simulink library "discreteGainScheduledFilteredPID"  (R2022a)
settings: Solver=VariableStepAuto  StartTime=0.0  StopTime=10.0  RelTol=1e-3
undefined symbols (not defined in the file): Ts
settings Model: Creator=adabney  LastModifiedBy=jacob

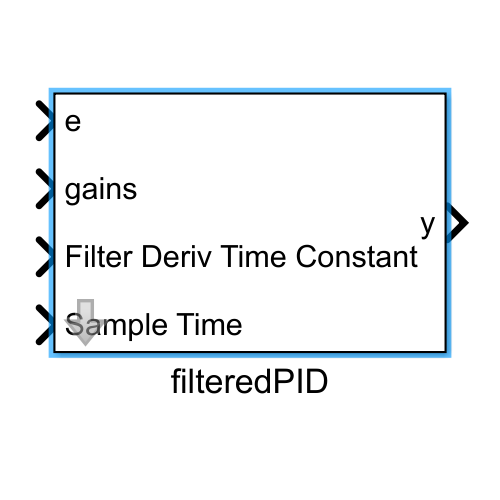
[thumbnail: Simulink's stored preview of the top-level diagram]
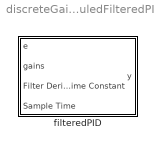
== system discreteGainScheduledFilteredPID ==
  filteredPID : Subsystem  mask{tau=0, Ts=Ts}
      mask prompts: tau "Filter Time Constant"; Ts "Sample Time"
      mask DialogControl DescTextVar Prompt: Gain-scheduled Discrete-time Filtered-PID Controller
      mask DialogControl ParameterGroupVar Prompt: Controller Inputs

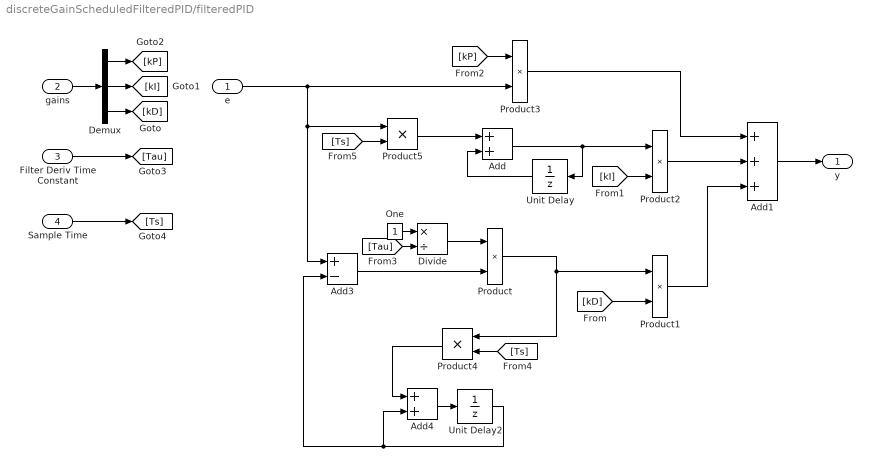
== system discreteGainScheduledFilteredPID/filteredPID ==
  e : Inport
  gains : Inport  Port=2
  Filter Deriv Time Constant : Inport  Port=3
  Sample Time : Inport  Port=4
  Add : Sum
  Add1 : Sum  Inputs=+++
  Add3 : Sum  Inputs=+-
  Add4 : Sum
  Demux : Demux  Outputs=3
  Divide : Product  Inputs=*/
  One : Constant  OutDataTypeStr=Inherit: Inherit via back propagation
  Product{,1..5} (6 alike) : Product
  Unit Delay : UnitDelay  SampleTime=-1  HasFrameUpgradeWarning=on
  Unit Delay2 : UnitDelay  SampleTime=-1  HasFrameUpgradeWarning=on
  y : Outport
  wires:
  Product1/1 -> Add1/3
  Product3/1 -> Add1/1
  [kD] -> Product1/2
  [kI] -> Product2/2
  [kP] -> Product3/1
  Add1/1 -> y/1
  Product2/1 -> Add1/2
  Add/1 -> Unit Delay/1, Product2/1
  Product/1 -> Product4/1, Product1/1
  gains/1 -> Demux/1
  Demux/1 -> [kP]
  Demux/2 -> [kI]
  Demux/3 -> [kD]
  Product5/1 -> Add/1
  Unit Delay/1 -> Add/2
  Product4/1 -> Add4/1
  e/1 -> Product3/2, Add3/1, Product5/1
  Add4/1 -> Unit Delay2/1
  Add3/1 -> Product/2
  Unit Delay2/1 -> Add4/2, Add3/2
  Filter Deriv Time Constant/1 -> [Tau]
  Sample Time/1 -> [Ts]
  One/1 -> Divide/1
  [Tau] -> Divide/2
  Divide/1 -> Product/1
  [Ts] -> Product4/2
  [Ts] -> Product5/2
